simulink model "model"  (R2020b)
settings: Solver=VariableStepAuto  StartTime=0.0  StopTime=10.0  RelTol=1e-3
undefined symbols (not defined in the file or in its folder): b, J, Kb, Kt, L, R
settings Model: Creator=Pavan  LastModifiedBy=Pavan

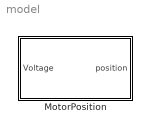
== system model ==
  MotorPosition : Subsystem

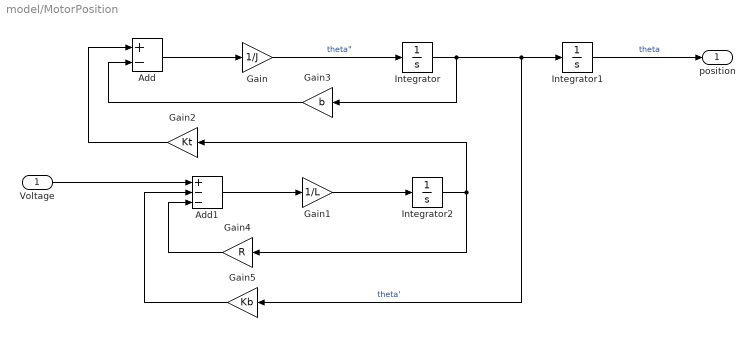
== system model/MotorPosition ==
  Voltage : Inport
  Add : Sum  Inputs=+-
  Add1 : Sum  Inputs=+--
  Gain : Gain  Gain=1/J
  Gain1 : Gain  Gain=1/L
  Gain2 : Gain  Gain=Kt
  Gain3 : Gain  Gain=b
  Gain4 : Gain  Gain=R
  Gain5 : Gain  Gain=Kb
  Integrator : Integrator
  Integrator1 : Integrator
  Integrator2 : Integrator
  position : Outport
  wires:
  Integrator/1 -> Gain3/1, Gain5/1, Integrator1/1  "theta'"
  Voltage/1 -> Add1/1
  Add/1 -> Gain/1
  Gain1/1 -> Integrator2/1
  Gain/1 -> Integrator/1  "theta\""
  Gain5/1 -> Add1/2
  Gain4/1 -> Add1/3
  Integrator1/1 -> position/1  "theta"
  Gain2/1 -> Add/1
  Integrator2/1 -> Gain4/1, Gain2/1
  Add1/1 -> Gain1/1
  Gain3/1 -> Add/2
